simulink model "PV_Single_Phase_inverter_afd_DC_AC"  (Simulink 8.3)
settings: Solver=ode45  StartTime=0.0  StopTime=0.7  RelTol=1e-3
undefined symbols (not defined in the file or in its folder): ln, Newton, Raphson
libraries: powerlib x13, powerlib_extras x3
settings Model: Creator=Birdman  LastModifiedBy=jt  SimulationMode=accelerator
settings OptimizationCC: InitFltsAndDblsToZero=on  EfficientMapNaN2IntZero=off
settings DebuggingCC: SaveWithParameterizedLinksMsg=none  SignalResolutionControl=TryResolveAllWithWarning  FcnCallInpInsideContextMsg=UseLocalSettings  StateNameClashWarn=none
settings HardwareCC: TargetIntDivRoundTo=Zero  TargetEndianess=LittleEndian  TargetHWDeviceType=MATLAB Host  ProdEqTarget=off
settings CodeAppCC: MaxIdLength=128

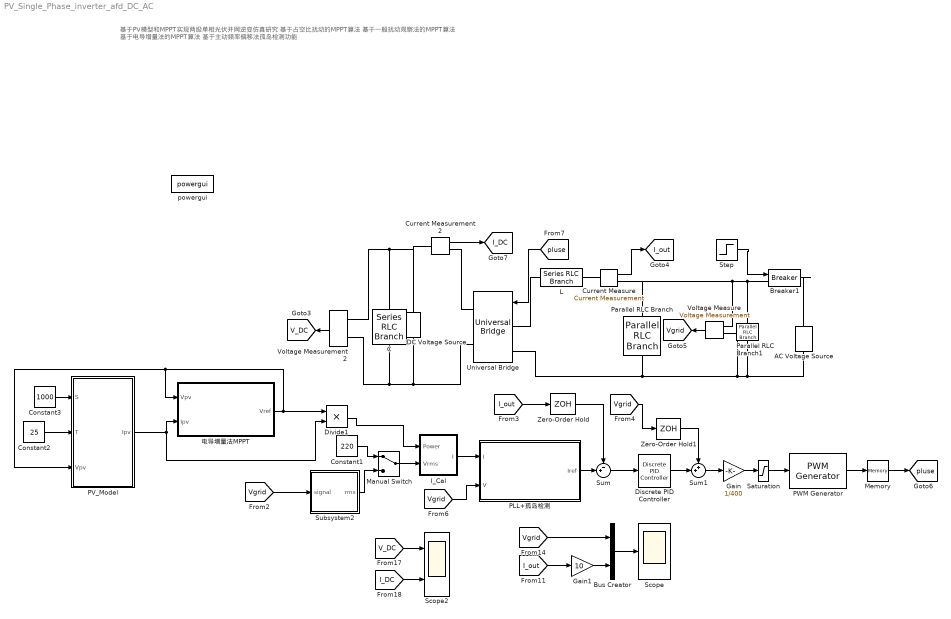
== system PV_Single_Phase_inverter_afd_DC_AC ==
  note: 基于PV模型和MPPT实现两级单相光伏并网逆变仿真研究
      | 基于占空比扰动的MPPT算法
      | 基于一般扰动观察法的MPPT算法
      | 基于电导增量法的MPPT算法
      | 基于主动频率偏移法孤岛检测功能
  AC Voltage Source : powerlib/Electrical Sources/AC Voltage Source  Amplitude=311  Phase=0  Frequency=50  SampleTime=0  Measurements=None
  Breaker1 : powerlib/Elements/Breaker  InitialState=1  SwitchingTimes="[ 1/60  5/60 ]"  External=on  BreakerResistance=0.01  SnubberResistance=1e5  SnubberCapacitance=inf  Measurements=None  MoreParameters=off  NoBreakLoop=off
  Bus Creator : BusCreator  Inputs=2
  C : powerlib/Elements/Series RLC Branch  LConnTagsString=__new0  RConnTagsString=__new0  BranchType=RC  Resistance=0.5  Inductance=22e-6  SetiL0=off  InitialCurrent=0  Capacitance=22e-6  Setx0=off  InitialVoltage=0  Measurements=None
  Constant1 : Constant  Value=220
  Constant2 : Constant  Value=25
  Constant3 : Constant  Value=1000
  Current Measure : powerlib/Measurements/Current Measurement  PhasorSimulation=off  OutputType=Complex  PSBequivalent=0
  Current Measurement2 : powerlib/Measurements/Current Measurement  PhasorSimulation=off  OutputType=Complex  PSBequivalent=0
  DC Voltage Source : powerlib/Electrical Sources/DC Voltage Source  Amplitude=500  Measurements=Voltage
  Discrete PID Controller : powerlib_extras/Discrete  Control Blocks/Discrete PID Controller  Kp=60  Ki=200  Kd=0  TcD=0.5e-3  Par_Limits=[1e6 -1e6]  Init=0  Ts=1e-4
  Divide1 : Product
  Gain : Gain  Gain=1/400
  Gain1 : Gain  Gain=10
  I_Cal : Subsystem
  L : powerlib/Elements/Series RLC Branch  LConnTagsString=__new0  RConnTagsString=__new0  BranchType=RL  Resistance=0.01  Inductance=6e-3  SetiL0=off  InitialCurrent=0  Capacitance=1e-6  Setx0=off  InitialVoltage=0  Measurements=None
  Manual Switch : ManualSwitch
  Memory : Memory
  PLL+孤岛检测 : Subsystem
      mask Display: disp('PLL+孤岛检测')
  PV_Model : Subsystem  mask{Vm=288, Im=13.88, Voc=354, Isc=14.88, Sref=1000, Tref=25, a=0.0025, b=0.0028, Rs=0.5}
      mask prompts: a "a(A/C)"; b "b(V/C)"
      mask Display: disp('PV_array')
  PWM Generator : powerlib_extras/Control  Blocks/PWM Generator  GeneratorMode="2-arm  bridge (4 pulses)"  Fc=1e4  Internal=off  mIndex=0.4  Freq=60  Phase=0
  Parallel RLC Branch : powerlib/Elements/Parallel RLC Branch  LConnTagsString=a  RConnTagsString=__new0  BranchType=RLC  Resistance=10.  Inductance=7.65e-3  SetiL0=off  InitialCurrent=0  Capacitance=1300e-6  Setx0=off  InitialVoltage=0  Measurements=None
  Parallel RLC Branch1 : powerlib/Elements/Parallel RLC Branch  LConnTagsString=a  RConnTagsString=__new0  BranchType=R  Resistance=100  Inductance=7.65e-3  SetiL0=off  InitialCurrent=0  Capacitance=1300e-6  Setx0=off  InitialVoltage=0  Measurements=None
  Saturation : Saturate  UpperLimit=0.99  LowerLimit=-0.99
  Scope : Scope
      settings: TimeRange=0.1  YMin=-350  YMax=300
  Scope2 : Scope  NumInputPorts=2
      settings: YMin=475~-2.5  YMax=525~35  SaveName=ScopeData3
  Step : Step  Time=0.2  Before=1  After=0  SampleTime=0
  Subsystem2 : Subsystem  mask{f=50}
      mask prompts: f "Fundamental frequency (Hz)"
      mask Display: disp('RMS')
  Sum : Sum  Inputs=-+|
  Sum1 : Sum  Inputs=++|
  Universal Bridge : powerlib/Power Electronics/Universal Bridge  Arms=2  SnubberResistance=1e5  SnubberCapacitance=inf  Device=IGBT / Diodes  Ron=1e-3  Lon=0  ForwardVoltages="[  0  0  ]"  ForwardVoltage=0  GTOparameters=[ 10e-6 , 20e-6 ]  IGBTparameters=[ 1e-6 , 2e-6 ]  Measurements=None  Measurements_2=None  converterType=Rectifier
  Voltage Measure : powerlib/Measurements/Voltage Measurement  PhasorSimulation=off  OutputType=Complex  PSBequivalent=0
  Voltage Measurement2 : powerlib/Measurements/Voltage Measurement  PhasorSimulation=off  OutputType=Complex  PSBequivalent=0
  Zero-Order Hold : ZeroOrderHold  SampleTime=1e-4
  Zero-Order Hold1 : ZeroOrderHold  SampleTime=1e-4
  powergui : powerlib/powergui  SimulationMode=Discrete  SolverType=Tustin  SampleTime=1e-6  frequency=60  SPID=off  DisableSnubberDevices=off  DisableRonSwitches=off  DisableVfSwitches=off  SwTol=0  Interpol=off  DisplayEquations=off  Ts=0  methode=off  frequencyindice=0  Pbase=100e6  ErrMax=1e-4  Iterations=50  UnitsV=kV  UnitsW=MW  FunctionMessages=off  echomessages=off  HookPort=off  EnableUseOfTLC=off  x0status=blocks  RestoreLinks=warning  ResistiveCurrentMeasurement=off  Frange=[0:2:500]  Ylog=off  Xlog=on  ShowGrid=off  save=off  variable=ZData  structure=io  ZoomFFT=off  StartTime=0.0  cycles=3  DisplayStyle=1  fundamental=50  FreqAxis=on  MaxFrequency=2500  frequencyindicesteady=1  RmsSteady=1  display=off
  电导增量法MPPT : Subsystem
      mask Display: disp('PV_array_MPPT')
  tag scope: I_DC=global, I_out=global, V_DC=global, Vgrid=global, pluse=global
  wires:
  Sum/1 -> Discrete PID Controller/1
  Sum1/1 -> Gain/1
  Discrete PID Controller/1 -> Sum1/2
  Zero-Order Hold1/1 -> Sum1/1
  Step/1 -> Breaker1/1
  PWM Generator/1 -> Memory/1
  Gain/1 -> Saturation/1
  Saturation/1 -> PWM Generator/1
  Zero-Order Hold/1 -> Sum/1
  Voltage Measurement2/1 -> [V_DC]
  Current Measure/1 -> [I_out]
  [I_out] -> Zero-Order Hold/1
  Voltage Measure/1 -> [Vgrid]
  [Vgrid] -> Zero-Order Hold1/1
  I_Cal/1(I) -> PLL+孤岛检测/1(I)
  PLL+孤岛检测/1(Iref) -> Sum/2
  [Vgrid] -> PLL+孤岛检测/2(V)
  Memory/1 -> [pluse]
  [pluse] -> Universal Bridge/1
  Bus Creator/1 -> Scope/1
  [I_out] -> Gain1/1
  [V_DC] -> Scope2/1
  Gain1/1 -> Bus Creator/2
  [I_DC] -> Scope2/2
  [Vgrid] -> Bus Creator/1
  Current Measurement2/1 -> [I_DC]
  Divide1/1 -> I_Cal/1(Power)
  Constant3/1 -> PV_Model/1(S)
  Constant2/1 -> PV_Model/2(T)
  电导增量法MPPT/1(Vref) -> Divide1/1, PV_Model/3(Vpv), 电导增量法MPPT/1(Vpv)
  PV_Model/1(Ipv) -> 电导增量法MPPT/2(Ipv), Divide1/2
  [Vgrid] -> Subsystem2/1(signal)
  Constant1/1 -> Manual Switch/1
  Subsystem2/1(rms) -> Manual Switch/2
  Manual Switch/1 -> I_Cal/2(Vrms)
  connections:
  Universal Bridge/LConn1 -- L/LConn1
  L/RConn1 -- Current Measure/LConn1
  Parallel RLC Branch/LConn1 -- Current Measure/RConn1 -- Parallel RLC Branch1/LConn1 -- Breaker1/LConn1 -- Voltage Measure/LConn1
  Breaker1/RConn1 -- AC Voltage Source/RConn1
  Universal Bridge/LConn2 -- Parallel RLC Branch/RConn1 -- Voltage Measure/LConn2 -- Parallel RLC Branch1/RConn1 -- AC Voltage Source/LConn1
  Voltage Measurement2/LConn1 -- DC Voltage Source/RConn1 -- Current Measurement2/LConn1 -- C/LConn1
  C/RConn1 -- Voltage Measurement2/LConn2 -- DC Voltage Source/LConn1 -- Universal Bridge/RConn2
  Current Measurement2/RConn1 -- Universal Bridge/RConn1

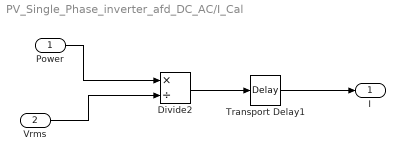
== system PV_Single_Phase_inverter_afd_DC_AC/I_Cal ==
  Power : Inport
  Vrms : Inport  Port=2
  Divide2 : Product  Inputs=*/
  Transport Delay1 : TransportDelay  DelayTime=1e-4
  I : Outport
  wires:
  Power/1 -> Divide2/1
  Vrms/1 -> Divide2/2
  Divide2/1 -> Transport Delay1/1
  Transport Delay1/1 -> I/1

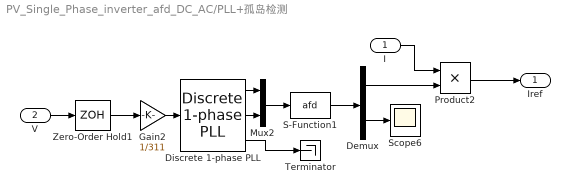
== system PV_Single_Phase_inverter_afd_DC_AC/PLL+孤岛检测 ==
  I : Inport
  V : Inport  Port=2
  Demux : Demux  Outputs=2
  Discrete 1-phase PLL : powerlib_extras/Discrete  Control Blocks/Discrete 1-phase PLL  Fmin=49.5  Par_Init=[0 50]  ParK="[150  100]"  Ts=1e-4  AGC=off
  Gain2 : Gain  Gain=1/311
  Mux2 : Mux  Inputs=2
  Product2 : Product  RndMeth=Zero
  S-Function1 : S-Function  FunctionName=afd  EnableBusSupport=off
  Scope6 : Scope
      settings: TimeRange=0.2  YMin=49.9895  YMax=50.0005  SaveName=freq
  Terminator : Terminator
  Zero-Order Hold1 : ZeroOrderHold  SampleTime=1e-4
  Iref : Outport
  wires:
  I/1 -> Product2/1
  S-Function1/1 -> Demux/1
  Discrete 1-phase PLL/1 -> Mux2/1
  Mux2/1 -> S-Function1/1
  Discrete 1-phase PLL/2 -> Mux2/2
  Gain2/1 -> Discrete 1-phase PLL/1
  Demux/1 -> Product2/2
  Demux/2 -> Scope6/1
  Discrete 1-phase PLL/3 -> Terminator/1
  Product2/1 -> Iref/1
  V/1 -> Zero-Order Hold1/1
  Zero-Order Hold1/1 -> Gain2/1

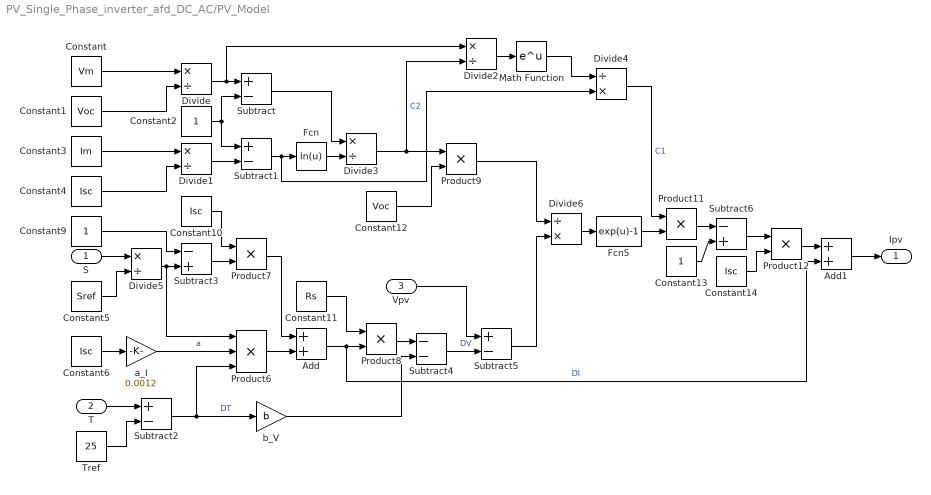
== system PV_Single_Phase_inverter_afd_DC_AC/PV_Model ==
  S : Inport
  T : Inport  Port=2
  Vpv : Inport  Port=3
  Add : Sum
  Add1 : Sum
  Constant : Constant  Value=Vm
  Constant1 : Constant  Value=Voc
  Constant{4,6,10,14} (4 alike) : Constant  Value=Isc
  Constant11 : Constant  Value=Rs
  Constant12 : Constant  Value=Voc
  Constant13 : Constant
  Constant2 : Constant
  Constant3 : Constant  Value=Im
  Constant5 : Constant  Value=Sref
  Constant9 : Constant
  Divide{,1..3,5} (5 alike) : Product  Inputs=*/
  Divide4 : Product  Inputs=/*
  Divide6 : Product  Inputs=/*
  Fcn : Fcn  Expr=ln(u)
  Fcn5 : Fcn  Expr=exp(u)-1
  Math Function : Math  SaturateOnIntegerOverflow=on
  Product{7..9,11..12} (5 alike) : Product  RndMeth=Zero
  Product6 : Product  Inputs=3  RndMeth=Zero
  Subtract{,1..2,5} (4 alike) : Sum  Inputs=+-
  Subtract3 : Sum  Inputs=-+
  Subtract4 : Sum  Inputs=--
  Subtract6 : Sum  Inputs=-+
  Tref : Constant  Value=25
  a_I : Gain  Gain=0.0012
  b_V : Gain  Gain=b
  Ipv : Outport
  wires:
  Constant1/1 -> Divide/2
  Constant/1 -> Divide/1
  Divide/1 -> Subtract/1, Divide2/1
  Constant2/1 -> Subtract/2, Subtract1/1
  Constant4/1 -> Divide1/2
  Constant3/1 -> Divide1/1
  Divide1/1 -> Subtract1/2
  Subtract1/1 -> Divide4/2, Fcn/1
  Subtract/1 -> Divide3/1
  Divide3/1 -> Product9/1, Divide2/2  "C2"
  Divide2/1 -> Math Function/1
  Math Function/1 -> Divide4/1
  Divide4/1 -> Product11/1  "C1"
  T/1 -> Subtract2/1
  Tref/1 -> Subtract2/2
  Subtract2/1 -> Product6/3, b_V/1  "DT"
  S/1 -> Divide5/1
  b_V/1 -> Subtract4/2
  Constant6/1 -> a_I/1
  a_I/1 -> Product6/2  "a"
  Divide5/1 -> Product6/1, Subtract3/2
  Constant9/1 -> Subtract3/1
  Subtract3/1 -> Product7/2
  Constant10/1 -> Product7/1
  Product7/1 -> Add/1
  Product6/1 -> Add/2
  Add/1 -> Product8/2, Add1/2  "DI"
  Constant11/1 -> Product8/1
  Product8/1 -> Subtract4/1
  Subtract4/1 -> Subtract5/2  "DV"
  Constant12/1 -> Product9/2
  Product9/1 -> Divide6/1
  Vpv/1 -> Subtract5/1
  Divide6/1 -> Fcn5/1
  Subtract5/1 -> Divide6/2
  Fcn5/1 -> Product11/2
  Product11/1 -> Subtract6/1
  Constant13/1 -> Subtract6/2
  Subtract6/1 -> Product12/1
  Constant14/1 -> Product12/2
  Product12/1 -> Add1/1
  Add1/1 -> Ipv/1
  Fcn/1 -> Divide3/2
  Constant5/1 -> Divide5/2

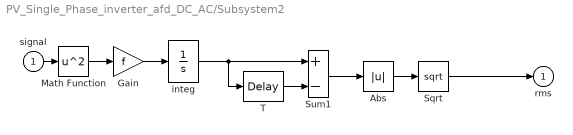
== system PV_Single_Phase_inverter_afd_DC_AC/Subsystem2 ==
  signal : Inport
  Abs : Abs  SaturateOnIntegerOverflow=on
  Gain : Gain  Gain=f  SaturateOnIntegerOverflow=on  OutDataTypeStr=Inherit: Same as input  ParamDataTypeStr=Inherit: Same as input
  Math Function : Math  Operator=square  SaturateOnIntegerOverflow=on
  Sqrt : Sqrt  AlgorithmType=Newton-Raphson  SaturateOnIntegerOverflow=on
  Sum1 : Sum  Inputs=+-  SaturateOnIntegerOverflow=on  InputSameDT=on  OutDataTypeStr=Inherit: Same as first input
  T : TransportDelay  DelayTime=1/f  BufferSize=2048
  integ : Integrator
  rms : Outport  InitialOutput=0
  wires:
  Sum1/1 -> Abs/1
  signal/1 -> Math Function/1
  Math Function/1 -> Gain/1
  Gain/1 -> integ/1
  T/1 -> Sum1/2
  Abs/1 -> Sqrt/1
  Sqrt/1 -> rms/1
  integ/1 -> T/1, Sum1/1

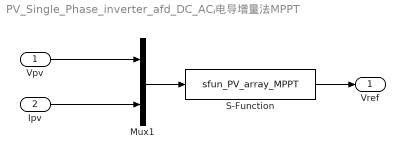
== system PV_Single_Phase_inverter_afd_DC_AC/电导增量法MPPT ==
  Vpv : Inport
  Ipv : Inport  Port=2
  Mux1 : Mux  Inputs=2
  S-Function : S-Function  FunctionName=sfun_PV_array_MPPT  EnableBusSupport=off
  Vref : Outport
  wires:
  S-Function/1 -> Vref/1
  Ipv/1 -> Mux1/2
  Mux1/1 -> S-Function/1
  Vpv/1 -> Mux1/1
